simulink model "Gep_Lab3_A2"  (R2020b)
settings: Solver=VariableStepAuto  StartTime=0.0  StopTime=0.2  MaxStep=10e-6  RelTol=10e-6
undefined symbols (not defined in the file): alpha, plecs
settings Model: Creator=barac  LastModifiedBy=barac

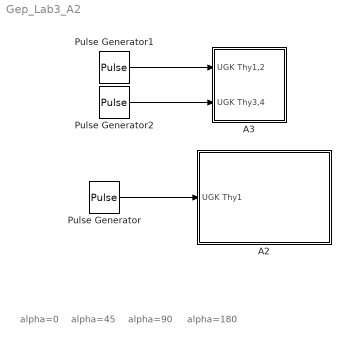
== system Gep_Lab3_A2 ==
  note: alpha=0
  note: alpha=45
  note: alpha=90
  note: alpha=180
  A2 : Subsystem  LoadFcn=plecs('sl', 200);  InitFcn=plecs('sl', 214);  StartFcn=plecs('sl', 208);  StopFcn=plecs('sl', 209);  mask(PlecsCircuit){PLECSData=<binary blob, 3120 chars, not shown>}
      mask prompts: PLECSData "PLECS Data (Do not delete or modify!)"
      mask init:
      | % PLACE CUSTOM INITIALIZATIONS ABOVE
      | % DO NOT REMOVE
      | plecs('sl', 215);
      | % DO NOT REMOVE
      settings: CopyFcn=plecs('sl', 203);  DeleteFcn=plecs('sl', 205);  UndoDeleteFcn=plecs('sl', 206);  PreSaveFcn=plecs('sl', 211);  PostSaveFcn=plecs('sl', 201);  NameChangeFcn=plecs('sl', 210);  DestroyFcn=plecs('sl', 207);  PreCopyFcn=plecs('sl', 216);  OpenFcn=plecs('sl', 202);  ErrorFcn=plerrorfcn
      mask Help: web(['file:///' fullfile(plecsdoc, 'creatingacircuit.html')])
      mask Display: disp('PLECS\nCircuit')
  A3 : Subsystem  LoadFcn=plecs('sl', 200);  InitFcn=plecs('sl', 214);  StartFcn=plecs('sl', 208);  StopFcn=plecs('sl', 209);  mask(PlecsCircuit){PLECSData=<binary blob, 4732 chars, not shown>}
      mask prompts: PLECSData "PLECS Data (Do not delete or modify!)"
      mask init:
      | % PLACE CUSTOM INITIALIZATIONS ABOVE
      | % DO NOT REMOVE
      | plecs('sl', 215);
      | % DO NOT REMOVE
      settings: CopyFcn=plecs('sl', 203);  DeleteFcn=plecs('sl', 205);  UndoDeleteFcn=plecs('sl', 206);  PreSaveFcn=plecs('sl', 211);  PostSaveFcn=plecs('sl', 201);  NameChangeFcn=plecs('sl', 210);  DestroyFcn=plecs('sl', 207);  PreCopyFcn=plecs('sl', 216);  OpenFcn=plecs('sl', 202);  ErrorFcn=plerrorfcn
      mask Help: web(['file:///' fullfile(plecsdoc, 'creatingacircuit.html')])
      mask Display: disp('PLECS\nCircuit')
  Pulse Generator : DiscretePulseGenerator  PulseType=Time based  Amplitude=230*sqrt(2)  Period=1/50  PhaseDelay=((1/50)/360)*alpha
  Pulse Generator1 : DiscretePulseGenerator  PulseType=Time based  Period=1/50  PulseWidth=5  PhaseDelay=((1/50)/360)*alpha
  Pulse Generator2 : DiscretePulseGenerator  PulseType=Time based  Period=1/50  PulseWidth=5  PhaseDelay=((1/50)/360)*alpha+0.01
  wires:
  Pulse Generator/1 -> A2/1(UGK Thy1)
  Pulse Generator1/1 -> A3/1(UGK Thy1,2)
  Pulse Generator2/1 -> A3/2(UGK Thy3,4)

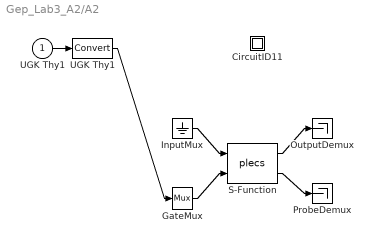
== system Gep_Lab3_A2/A2 ==
  UGK Thy1 : Inport  PortDimensions=1
  " CircuitID11 " : Subsystem
  " GateMux " : Mux  Inputs=[ 1 ]
  " InputMux " : Ground
  " OutputDemux " : Terminator
  " ProbeDemux " : Terminator
  " S-Function " : S-Function  FunctionName=plecs  SFunctionDeploymentMode=off  EnableBusSupport=off
  " UGK Thy1 " : DataTypeConversion  SaturateOnIntegerOverflow=on  RndMeth=Zero
  wires:
  " InputMux "/1 -> " S-Function "/1
  " GateMux "/1 -> " S-Function "/2
  " S-Function "/1 -> " OutputDemux "/1
  " S-Function "/2 -> " ProbeDemux "/1
  UGK Thy1/1 -> " UGK Thy1 "/1
  " UGK Thy1 "/1 -> " GateMux "/1

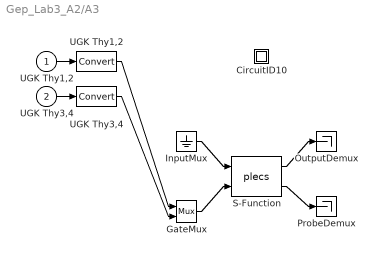
== system Gep_Lab3_A2/A3 ==
  UGK Thy1,2 : Inport  PortDimensions=1
  UGK Thy3,4 : Inport  Port=2  PortDimensions=1
  " CircuitID10 " : Subsystem
  " GateMux " : Mux  Inputs=[ 1 1 ]
  " InputMux " : Ground
  " OutputDemux " : Terminator
  " ProbeDemux " : Terminator
  " S-Function " : S-Function  FunctionName=plecs  SFunctionDeploymentMode=off  EnableBusSupport=off
  " UGK Thy1,2 " : DataTypeConversion  SaturateOnIntegerOverflow=on  RndMeth=Zero
  " UGK Thy3,4 " : DataTypeConversion  SaturateOnIntegerOverflow=on  RndMeth=Zero
  wires:
  " InputMux "/1 -> " S-Function "/1
  " GateMux "/1 -> " S-Function "/2
  " S-Function "/1 -> " OutputDemux "/1
  " S-Function "/2 -> " ProbeDemux "/1
  UGK Thy1,2/1 -> " UGK Thy1,2 "/1
  " UGK Thy1,2 "/1 -> " GateMux "/1
  UGK Thy3,4/1 -> " UGK Thy3,4 "/1
  " UGK Thy3,4 "/1 -> " GateMux "/2

== system Gep_Lab3_A2/A2/ CircuitID11  ==

== system Gep_Lab3_A2/A3/ CircuitID10  ==
